simulink model "problem4"  (R2020b)
settings: Solver=VariableStepAuto  StartTime=0.0  StopTime=0.1  RelTol=1e-3
values from neighbouring files (symbols this model uses):
  b = 3.5077E-6    [prob4_data.sldd]
  J = 3.2284E-6    [prob4_data.sldd]
  Ke = 0.0274    [prob4_data.sldd]
  Kt = 0.0274    [prob4_data.sldd]
  L = 2.75E-6    [prob4_data.sldd]
  R = 4.0    [prob4_data.sldd]
settings Model: DataDictionary=prob4_data.sldd  Creator=Varun  LastModifiedBy=Varun

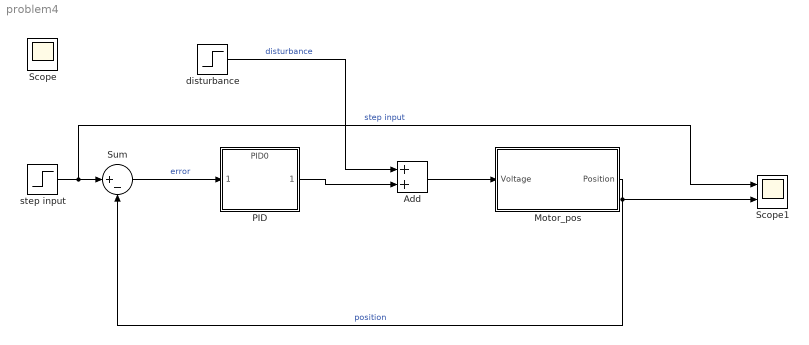
== system problem4 ==
  Add : Sum
  Motor_pos : Subsystem
  PID : ModelReference  ModelNameDialog=PID0  SimulationMode=Normal  ModelReferenceVersion=1.9
  Scope1 : Scope  NumInputPorts=2
  Sum : Sum  Inputs=|+-
  disturbance : Step  Time=0.02  SampleTime=0
  step input : Step  Time=0  SampleTime=0
  Scope : Scope
  wires:
  step input/1 -> Scope1/1, Sum/1  "step input"
  Sum/1 -> PID/1  "error"
  PID/1 -> Add/2
  disturbance/1 -> Add/1  "disturbance"
  Add/1 -> Motor_pos/1(Voltage)
  Motor_pos/1(Position) -> Scope1/2, Sum/2  "position"

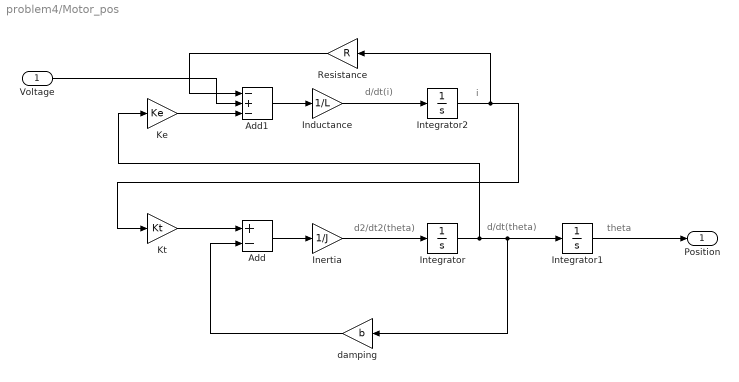
== system problem4/Motor_pos ==
  note: i
  note: d/dt(i)
  note: d2/dt2(theta)
  note: d/dt(theta)
  note: theta
  Voltage : Inport
  Add : Sum  Inputs=+-
  Add1 : Sum  Inputs=-+-
  Inductance : Gain  Gain=1/L
  Inertia : Gain  Gain=1/J
  Integrator : Integrator
  Integrator1 : Integrator
  Integrator2 : Integrator
  Ke : Gain  Gain=Ke
  Kt : Gain  Gain=Kt
  Resistance : Gain  Gain=R
  damping : Gain  Gain=b
  Position : Outport
  wires:
  Integrator1/1 -> Position/1
  Add1/1 -> Inductance/1
  damping/1 -> Add/2
  Resistance/1 -> Add1/1
  Ke/1 -> Add1/3
  Voltage/1 -> Add1/2
  Inductance/1 -> Integrator2/1
  Integrator/1 -> Integrator1/1, damping/1, Ke/1
  Kt/1 -> Add/1
  Add/1 -> Inertia/1
  Integrator2/1 -> Kt/1, Resistance/1
  Inertia/1 -> Integrator/1
